simulink subsystem "ElectricMachine3SSC"  (R2023b)
settings: Solver=VariableStepAuto  StartTime=0.0  StopTime=10.0  RelTol=1e-3
undefined symbols (not defined in the file): EnvAirTemp, PlntEM3EffTbl
libraries: fl_lib x5, nesl_utility_internal x4, ee_lib x1
settings Model: Creator=The MathWorks, Inc.  LastModifiedBy=The MathWorks, Inc.
settings OptimizationCC: ReuseModelBlockBuffer=off

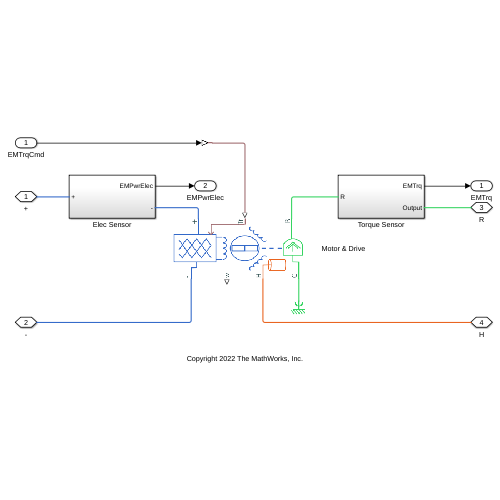
[thumbnail: Simulink's stored preview of the top-level diagram]
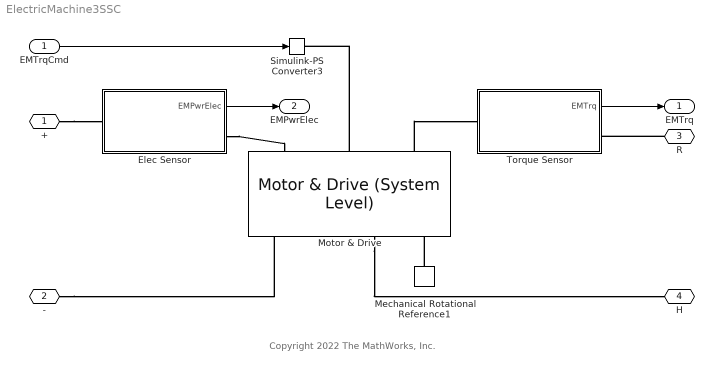
== system ElectricMachine3SSC ==
  note: Copyright 2022 The MathWorks, Inc.
  EMTrqCmd : Inport
  Elec Sensor : Subsystem
  Mechanical Rotational Reference1 : fl_lib/Mechanical/Rotational Elements/Mechanical Rotational Reference
  Motor & Drive : ee_lib/Electromechanical/Motor & Drive (System Level)  torque_speed_param=ee.enum.electromech.envelope.tabulated  overtorque_param=ee.enum.electromech.overtorque.no  T_t=PlntEM3Trq N*m  T_t_intermittent=[.36, .32, .28, 0] N*m  T_t_2D=[.09, .09, .09; .08, .08, .08; .07, .07, .07; 0, 0, 0] N*m  T_t_intermittent_2D=[.36, .36, .36; .32, .32, .32; .28, .28, .28; 0, 0, 0] N*m  w_t=PlntEM3Spd rad/s  vdc_t=[6, 12, 24] V  torque_max=0.1 N*m  power_max=30 W  torque_max_intermittent=0.4 N*m  power_max_intermittent=120 W  time_overtorque=30 s  time_recover=60 s  Tc=PlntEM3TimeCnst s  EnableSwitch=simscape.enum.onoff.off  losses_param=3  eff=100  w_eff=3750 rpm  T_eff=0.08 N*m  Piron=0 W  Pbase=0 W  w_eff_vec=PlntEM3Spd rad/s  T_eff_vec=PlntEM3TrqEff N*m  v_eff_vec=[100, 250, 400] V  losses_mat=[1.49, 1.67, 2.21, 3.1; .42, .69, 1.14, 2.03; .06, .24, .78, 1.68; .42, .69, 1.14, 2.03; 1.49, 1.67, 2.21, 3.1] W  efficiency_mat=PlntEM3EffTbl  losses_mat_3D=ones(5, 4, 3) W  efficiency_mat_3D=95 * ones(5, 4, 3)  Res=PlntEM3ExtSplySerRes Ohm  enable_fault=simscape.enum.onoff.off  fault_condition=1  fault_threshold=0.5  J=0 %EM Inertia accounted for in Drivetrain kg*m^2  lam=PlntEM3RotDamp N*m/(rad/s)  speed0=PlntEM3RotInitSpd rad/s  faulted_specify=off  faulted_priority=None  faulted=0  faulted_nominal_specify=off  faulted_nominal_unit=1  faulted_nominal_value=1  isSwitchedOff_specify=off  isSwitchedOff_priority=None  isSwitchedOff=0  isSwitchedOff_nominal_specify=off  isSwitchedOff_nominal_unit=1  isSwitchedOff_nominal_value=1  torqueLimitContinuous_specify=off  torqueLimitContinuous_priority=None  torqueLimitContinuous=0 N*m  torqueLimitContinuous_nominal_specify=off  torqueLimitContinuous_nominal_unit=N*m  torqueLimitContinuous_nominal_value=1  alpha=3.93e-3 1/K  Tmeas=EnvAirTemp K  Tmeas2=EnvAirTemp+100 K  losses_mat_T2=[1.49, 1.74, 2.49, 3.74; .42, .67, 1.42, 2.67; .06, .31, 1.06, 2.31; .42, .67, 1.42, 2.67; 1.49, 1.74, 2.49, 3.74] W  efficiency_mat_T2=0.8*PlntEM3EffTbl  losses_mat_3D_T2=ones(5, 4, 3) W  efficiency_mat_3D_T2=95 * ones(5, 4, 3)  thermal_mass=100 J/K  initial_temperature=EnvAirTemp K
      settings: InternalSimscapePortConfiguration="{\"Bottom\":[],\"Left\":[{\"id\":\"Vp\",\"label\":\"+\",\"type\":\"foundation.electrical.electrical\"},{\"id\":\"Tr\",\"label\":\"Tr\",\"type\":\"input\"},{\"id\":\"R\",\"label\":\"R\",\"type\":\"foundation.mechanical.rotational.rotational\"}],\"Right\":[{\"id\":\"Vm\",\"label\":\"-\",\"type\":\"foundation.electrical.electrical\"},{\"id\":\"Omega\",\"label\":\"w\",\"type\":\"output\"},{\"id\":\"H\",\"label\":\"H\",\"type\":\"foundation.thermal.thermal\"},{\"id\":\"C\",\"label\":\"C\",\"type\":\"foundation.mechanical.rotational.rotational\"}],\"Top\":[]}"
  Simulink-PS Converter3 : nesl_utility_internal/Simulink-PS Converter  PhysicalDomain=network_engine_domain  SubClassName=ps_input  LeftPortType=input  RightPortType=output  PseudoPeriodic=off  Frequencies=[]  NoiseDistribution=none  NoiseParameters=[]  Unit=N*m  AffineConversion=off  FilteringAndDerivatives=provide  SimscapeFilterOrder=1  InputFilterTimeConstant=0.001  UdotUserProvided=0
  Torque Sensor : Subsystem
  + : PMIOPort  Side=Left
  - : PMIOPort  Port=2  Side=Left
  R : PMIOPort  Port=3  Side=Right
  H : PMIOPort  Port=4  Side=Right
  EMTrq : Outport  VectorParamsAs1DForOutWhenUnconnected=off
  EMPwrElec : Outport  Port=2
  wires:
  Elec Sensor/1(EMPwrElec) -> EMPwrElec/1
  Torque Sensor/1(EMTrq) -> EMTrq/1
  EMTrqCmd/1 -> Simulink-PS Converter3/1
  connections:
  R/RConn1 -- Torque Sensor/RConn1
  Motor & Drive/LConn2 -- Simulink-PS Converter3/RConn1
  -/RConn1 -- Motor & Drive/RConn1
  +/RConn1 -- Elec Sensor/LConn1
  Elec Sensor/RConn1 -- Motor & Drive/LConn1
  Motor & Drive/LConn3 -- Torque Sensor/LConn1
  Mechanical Rotational Reference1/LConn1 -- Motor & Drive/RConn4
  Motor & Drive/RConn3 -- H/RConn1

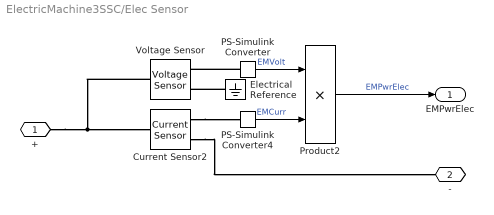
== system ElectricMachine3SSC/Elec Sensor ==
  Current Sensor2 : fl_lib/Electrical/Electrical Sensors/Current Sensor
  Electrical Reference : fl_lib/Electrical/Electrical Elements/Electrical Reference
  PS-Simulink Converter : nesl_utility_internal/PS-Simulink Converter  PhysicalDomain=network_engine_domain  SubClassName=ps_output  LeftPortType=input  RightPortType=output  PseudoPeriodic=off  Frequencies=[]  VectorFormat=1-D array  Unit=inherit  AffineConversion=off
  PS-Simulink Converter4 : nesl_utility_internal/PS-Simulink Converter  PhysicalDomain=network_engine_domain  SubClassName=ps_output  LeftPortType=input  RightPortType=output  PseudoPeriodic=off  Frequencies=[]  VectorFormat=1-D array  Unit=1  AffineConversion=off
  Product2 : Product
  Voltage Sensor : fl_lib/Electrical/Electrical Sensors/Voltage Sensor
  + : PMIOPort  Side=Left
  - : PMIOPort  Port=2  Side=Right
  EMPwrElec : Outport
  wires:
  PS-Simulink Converter4/1 -> Product2/2  "EMCurr"
  Product2/1 -> EMPwrElec/1  "EMPwrElec"
  PS-Simulink Converter/1 -> Product2/1  "EMVolt"
  connections:
  Current Sensor2/RConn1 -- PS-Simulink Converter4/LConn1
  Current Sensor2/RConn2 -- -/RConn1
  +/RConn1 -- Voltage Sensor/LConn1 -- Current Sensor2/LConn1
  Electrical Reference/LConn1 -- Voltage Sensor/RConn2
  PS-Simulink Converter/LConn1 -- Voltage Sensor/RConn1

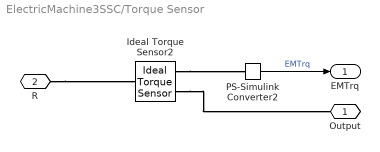
== system ElectricMachine3SSC/Torque Sensor ==
  Ideal Torque Sensor2 : fl_lib/Mechanical/Mechanical Sensors/Ideal Torque Sensor
  PS-Simulink Converter2 : nesl_utility_internal/PS-Simulink Converter  PhysicalDomain=network_engine_domain  SubClassName=ps_output  LeftPortType=input  RightPortType=output  PseudoPeriodic=off  Frequencies=[]  VectorFormat=1-D array  Unit=1  AffineConversion=off
  Output : PMIOPort  Side=Right
  R : PMIOPort  Port=2  Side=Left
  EMTrq : Outport
  wires:
  PS-Simulink Converter2/1 -> EMTrq/1  "EMTrq"
  connections:
  Ideal Torque Sensor2/RConn2 -- PS-Simulink Converter2/LConn1
  R/RConn1 -- Ideal Torque Sensor2/LConn1
  Ideal Torque Sensor2/RConn1 -- Output/RConn1
